simulink model "MotionControl"  (R2022a)
settings: Solver=VariableStepAuto  StartTime=0.0  StopTime=10.0  RelTol=1e-3
settings Model: Creator=Jakob  LastModifiedBy=Jakob

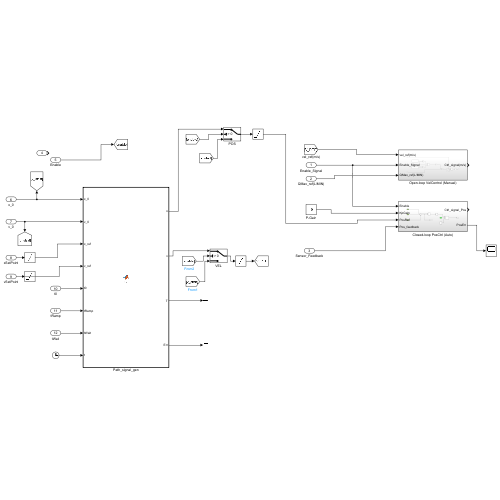
[thumbnail: Simulink's stored preview of the top-level diagram]
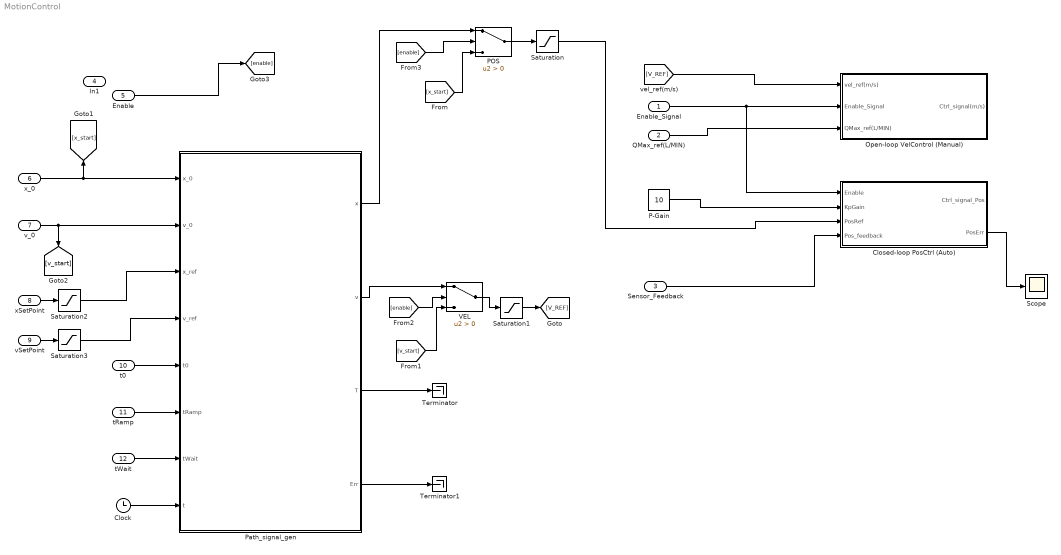
== system MotionControl ==
  Enable_Signal : Inport
  QMax_ref(L/MIN) : Inport  Port=2
  Sensor_Feedback : Inport  Port=3
  In1 : Inport  Port=4
  Enable : Inport  Port=5
  x_0 : Inport  Port=6
  v_0 : Inport  Port=7
  xSetPoint : Inport  Port=8
  vSetPoint : Inport  Port=9
  t0 : Inport  Port=10
  tRamp : Inport  Port=11
  tWait : Inport  Port=12
  Clock : Clock
  Closed-loop PosCtrl (Auto) : Subsystem
  Open-loop VelControl (Manual) : Subsystem
  P-Gain : Constant  Value=10
  POS : Switch  Criteria=u2 > Threshold  SaturateOnIntegerOverflow=off  InputSameDT=off
  Path_signal_gen : MATLAB Function  TreatAsAtomicUnit=on
  Saturation : Saturate
  Saturation1 : Saturate
  Saturation2 : Saturate
  Saturation3 : Saturate  UpperLimit=0.05  LowerLimit=-0.05
  Scope : Scope
  Terminator : Terminator
  Terminator1 : Terminator
  VEL : Switch  Criteria=u2 > Threshold  SaturateOnIntegerOverflow=off  InputSameDT=off
  wires:
  [V_REF] -> Open-loop VelControl (Manual)/1(vel_ref(m/s))
  Enable_Signal/1 -> Closed-loop PosCtrl (Auto)/1(Enable), Open-loop VelControl (Manual)/2(Enable_Signal)
  QMax_ref(L/MIN)/1 -> Open-loop VelControl (Manual)/3(QMax_ref(L/MIN))
  Closed-loop PosCtrl (Auto)/2(PosErr) -> Scope/1
  Clock/1 -> Path_signal_gen/8(t)
  P-Gain/1 -> Closed-loop PosCtrl (Auto)/2(KpGain)
  Sensor_Feedback/1 -> Closed-loop PosCtrl (Auto)/4(Pos_feedback)
  tWait/1 -> Path_signal_gen/7(tWait)
  tRamp/1 -> Path_signal_gen/6(tRamp)
  t0/1 -> Path_signal_gen/5(t0)
  vSetPoint/1 -> Saturation3/1
  xSetPoint/1 -> Saturation2/1
  v_0/1 -> [v_start], Path_signal_gen/2(v_0)
  x_0/1 -> Path_signal_gen/1(x_0), [x_start]
  Path_signal_gen/2(v) -> VEL/1
  Path_signal_gen/1(x) -> POS/1
  Enable/1 -> [enable]
  POS/1 -> Saturation/1
  VEL/1 -> Saturation1/1
  Saturation/1 -> Closed-loop PosCtrl (Auto)/3(PosRef)
  Saturation1/1 -> [V_REF]
  Path_signal_gen/4(Err) -> Terminator1/1
  Path_signal_gen/3(T) -> Terminator/1
  [x_start] -> POS/3
  [v_start] -> VEL/3
  [enable] -> VEL/2
  [enable] -> POS/2
  Saturation2/1 -> Path_signal_gen/3(x_ref)
  Saturation3/1 -> Path_signal_gen/4(v_ref)

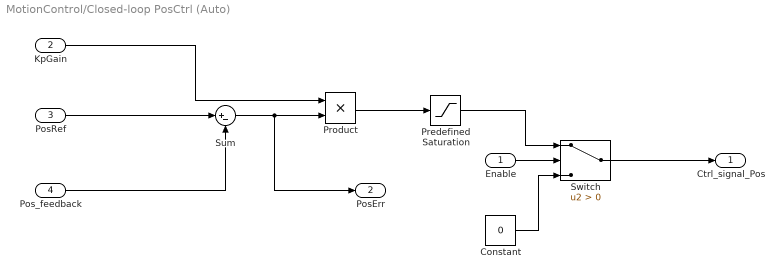
== system MotionControl/Closed-loop PosCtrl (Auto) ==
  Enable : Inport
  KpGain : Inport  Port=2
  PosRef : Inport  Port=3
  Pos_feedback : Inport  Port=4
  Constant : Constant  Value=0
  Predefined Saturation : Saturate  UpperLimit=1  LowerLimit=-1
  Product : Product
  Sum : Sum  Inputs=|+-
  Switch : Switch  Criteria=u2 > Threshold  SaturateOnIntegerOverflow=off  InputSameDT=off
  Ctrl_signal_Pos : Outport
  PosErr : Outport  Port=2
  wires:
  PosRef/1 -> Sum/1
  Pos_feedback/1 -> Sum/2
  Sum/1 -> PosErr/1, Product/2
  KpGain/1 -> Product/1
  Product/1 -> Predefined Saturation/1
  Predefined Saturation/1 -> Switch/1
  Switch/1 -> Ctrl_signal_Pos/1
  Enable/1 -> Switch/2
  Constant/1 -> Switch/3

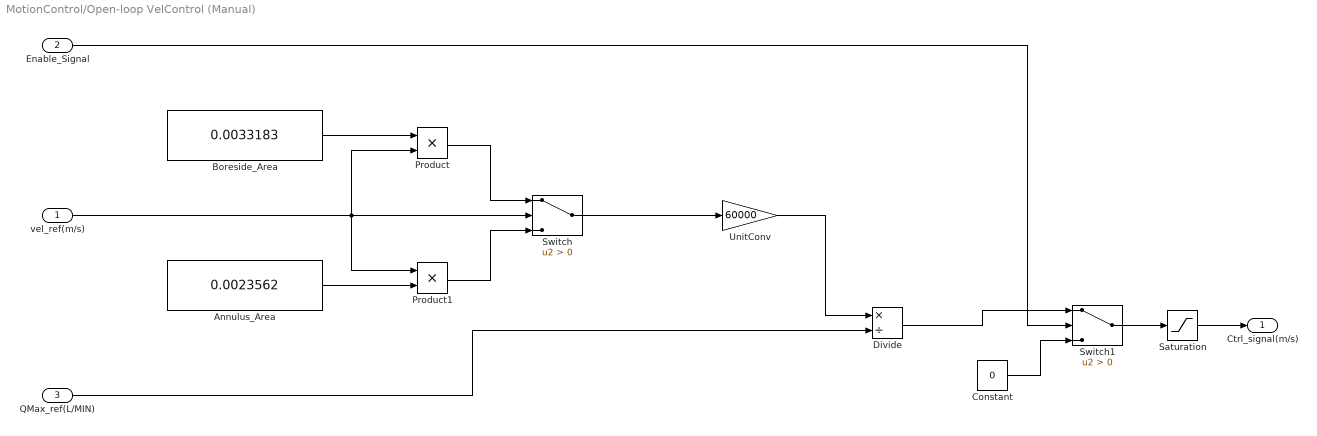
== system MotionControl/Open-loop VelControl (Manual) ==
  vel_ref(m/s) : Inport
  Enable_Signal : Inport  Port=2
  QMax_ref(L/MIN) : Inport  Port=3
  Annulus_Area : Constant  Value=0.0023562
  Boreside_Area : Constant  Value=0.0033183
  Constant : Constant  Value=0
  Divide : Product  Inputs=*/
  Product : Product
  Product1 : Product
  Saturation : Saturate  UpperLimit=0.05  LowerLimit=-0.05
  Switch : Switch  Criteria=u2 > Threshold  SaturateOnIntegerOverflow=off  InputSameDT=off
  Switch1 : Switch  Criteria=u2 > Threshold  SaturateOnIntegerOverflow=off  InputSameDT=off
  UnitConv : Gain  Gain=60000
  Ctrl_signal(m/s) : Outport
  wires:
  Divide/1 -> Switch1/1
  UnitConv/1 -> Divide/1
  Constant/1 -> Switch1/3
  Switch/1 -> UnitConv/1
  Enable_Signal/1 -> Switch1/2
  Product1/1 -> Switch/3
  Product/1 -> Switch/1
  vel_ref(m/s)/1 -> Product1/1, Product/2, Switch/2
  Boreside_Area/1 -> Product/1
  Annulus_Area/1 -> Product1/2
  QMax_ref(L/MIN)/1 -> Divide/2
  Switch1/1 -> Saturation/1
  Saturation/1 -> Ctrl_signal(m/s)/1

== matlab function MotionControl/Path_signal_gen ==
  data: x_0 input; v_0 input; x_ref input; v_ref input; t0 input; tRamp input; tWait input; t input; x output; v output; T output; Err output
function [x, v, T, Err]= fcn(x_0, v_0, x_ref, v_ref, t0, tRamp, tWait, t)

x_SetPoint = x_ref - x_0;
vs = v_ref; 
slopeExt = v_0-vs;
slopeRetr = -vs-v_0; 

as = vs/tRamp; % Find acceleration
s_acc = (vs^2-v_0^2)/as; % Acceleration sp

tHold = (x_SetPoint-s_acc)/vs;

if tHold < 0
    Err = 1;
else
    Err = 0;
end 

t1 = tRamp;
t2 = tHold;
t3 = tRamp;
t4 = tWait;
t5 = t1;
t6 = t2;
t7 = t3; 

% Equations of motion:
x1 = x0 + v_0*((t0+t1)-t0) - (slopeExt/t1)*((t0+t1)-t0)^2/2; 
x2 = x1 + vs * ((t0+t1+t2)-(t0+t1)); 
x4 = x_ref - v_0 * ((t0+t1+t2+t3+t4+t5)-(t0+t1+t2+t3+t4)) + (slopeRetr/t5)*((t0+t1+t2+t3+t4+t5)-(t0+t1+t2+t3+t4))^2/2; 
x5 = x4 - vs*((t0+t1+t2+t3+t4+t5+t6)-(t0+t1+t2+t3+t4+t5)); 

if Error == 1
    x = x0;
    v = v_0;
elseif t >= 0 && t<t0
    x = x0;
    v = v_0;
elseif t >= t0 && t < (t0+t1)
    x = x0 + v_0*(t-t0) - (slopeExt/t1)*(t-t0)^2/2;
    v = v_0 - (slopeExt/t1)*(t-t0); 
elseif t >=(t0+t1) && t < (t0+t1+t2)
    x = x1 + vs*(t-(t0+t1));
    v = vs;
elseif t>=(t0+t1+t2) && t<(t0+t1+t2+t3)
    x = x2 + vs*(t-(t0+t1+t2)) + (slopeExt/t3)*(t-(t0+t1+t2))^2/2;
    v = vs + (slopeExt/t3)*(t-(t0+t1+t2)); 
elseif t >=(t0+t1+t2+t3) && t<(t0+t1+t2+t3+t4)
    x = x_ref;
    v = v_0;
elseif t>=(t0+t1+t2+t3+t4) && t < (t0+t1+t2+t3+t4+t5)
    x = x_ref - v_0*(t-(t0+t1+t2+t3+t4))+(slopeRetr/t5)*(t-(t0+t1+t2+t3+t4))^2/2;
    v = v_0 + (slopeRetr/t5)*(t-(t0+t1+t2+t3+t4)); 
elseif t>=(t0+t1+t2+t3+t4+t5) && t < (t0+t1+t2+t3+t4+t5+t6)
    x = x4 - vs*(t-(t0+t1+t2+t3+t4+t5));
    v = -vs;
elseif t >= (t0+t1+t2+t3+t4+t5+t6) && t < (t0+t1+t2+t3+t4+t5+t6+t7)
    x = x5 - vs*(t-(t0+t1+t2+t3+t4+t5+t6)) - (slopeRetr/t3)*(t-(t0+t1+t2+t3+t4+t5+t6))^2/2;
    v = -vs-(slopeRetr/t3)*(t-(t0+t1+t2+t3+t4+t5+t6));
else
    x = x0;
    v = v0;
end 

T = t0+t1+t2+t3+t4+t5+t6+t7;
